simulink model "Task24"  (R2025a)
settings: Solver=VariableStepAuto  StartTime=0.0  StopTime=10.0  RelTol=1e-3
libraries: simulink x1
settings Model: Creator=LOQ  LastModifiedBy=LOQ

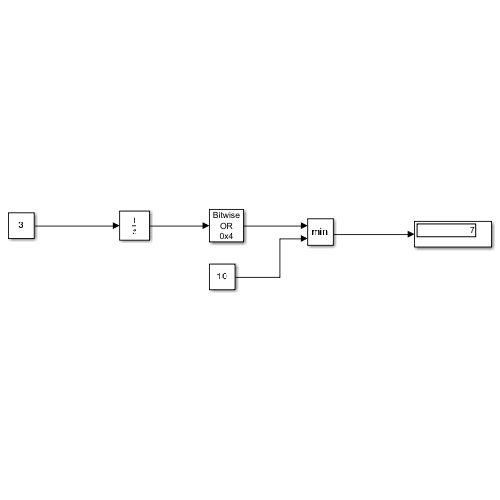
[thumbnail: Simulink's stored preview of the top-level diagram]
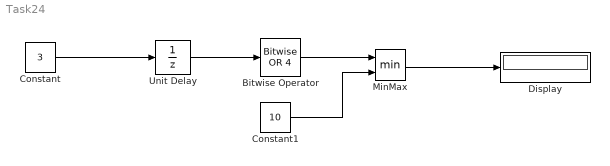
== system Task24 ==
  Bitwise Operator : simulink/Logic and Bit Operations/Bitwise Operator  logicop=OR  UseBitMask=on  BitMask=4  BitMaskRealWorld=Stored Integer
  Constant : Constant  Value=3  OutDataTypeStr=uint8
  Constant1 : Constant  Value=10  OutDataTypeStr=uint8
  Display : Display
  MinMax : MinMax  Inputs=2
  Unit Delay : UnitDelay  SampleTime=-1  HasFrameUpgradeWarning=on
  wires:
  Constant/1 -> Unit Delay/1
  Unit Delay/1 -> Bitwise Operator/1
  Bitwise Operator/1 -> MinMax/1
  Constant1/1 -> MinMax/2
  MinMax/1 -> Display/1
